simulink model "M2_chart_2"  (R2024a)
settings: Solver=FixedStepDiscrete  StartTime=0.0  StopTime=10.0  FixedStep=0.01  RelTol=1e-3  EnableMultiTasking=on
settings Model: Creator=saura  LastModifiedBy=Ishant
settings SolverCC: AlgebraicLoopSolver=TrustRegion  AutoInsertRateTranBlk=on
settings DataIOCC: LimitDataPoints=on
settings OptimizationCC: LifeSpan=inf
settings DebuggingCC: UnconnectedInputMsg=warning  UnconnectedOutputMsg=warning  UnconnectedLineMsg=warning  AllowSymbolicDim=off  SFUnexpectedBacktrackingDiag=warning  SFNoUnconditionalDefaultTransitionDiag=warning  SFExecutionAtInitializationDiag=none  ArithmeticOperatorsInVariantConditions=warning
settings ModelReferenceCC: EnableRefExpFcnMdlSchedulingChecks=on
settings SFSimCC: SimUseLocalCustomCode=off  CustomCodeUndefinedFunction=UseInterfaceOnly
settings RTWCC: RTWUseLocalCustomCode=off  GPUComputeCapability=3.5  DLArmComputeVersion=19.05
settings CodeAppCC: StateflowObjectComments=on
settings GRTTargetCC: TargetLangStandard=C89/C90 (ANSI)
settings ConfigComp: CovMetricSettings=dw  CovSaveCumulativeToWorkspaceVar=on  CovSaveSingleToWorkspaceVar=on  CovExternalEMLEnable=off  CovSFcnEnable=off

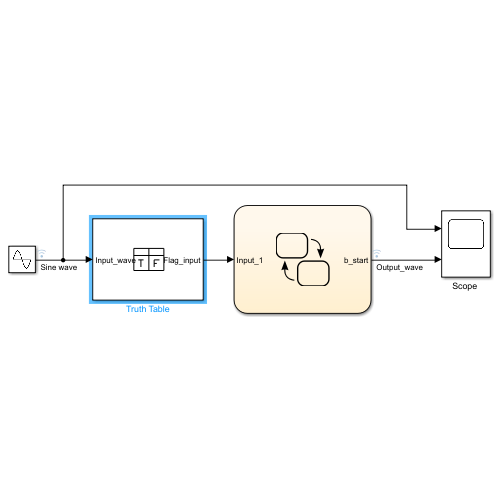
[thumbnail: Simulink's stored preview of the top-level diagram]
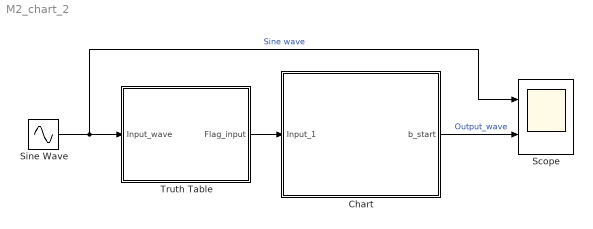
== system M2_chart_2 ==
  Chart : Stateflow chart  TreatAsAtomicUnit=on
  "Scope " : Scope  NumInputPorts=2
  Sine Wave : Sin  Amplitude=0.6
  Truth Table : Truth Table  TreatAsAtomicUnit=on
  wires:
  Sine Wave/1 -> "Scope "/1, Truth Table/1(Input_wave)  "Sine wave"
  Truth Table/1(Flag_input) -> Chart/1(Input_1)
  Chart/1(b_start) -> "Scope "/2  "Output_wave"

== matlab function M2_chart_2/Truth Table ==
  data: Input_wave input; Flag_input output
function Flag_input = fcn(Input_wave)

aVarTruthTableCondition_1 = false;
aVarTruthTableCondition_2 = false;


% condition2

aVarTruthTableCondition_1 = logical(Input_wave<=0.5);

% condition 1

aVarTruthTableCondition_2 = logical(Input_wave >0.5);

if (aVarTruthTableCondition_2)
    aFcnTruthTableAction_2();
elseif (aVarTruthTableCondition_1)
    aFcnTruthTableAction_1();
else % Default
    aFcnTruthTableAction_3();
end

function aFcnTruthTableAction_1()

% Example action 1 called from D2 column in condition table

Flag_input = 1;

function aFcnTruthTableAction_2()

% Example action 2 called from D1 column in condition table

Flag_input = -1

function aFcnTruthTableAction_3()

% nothing

Flag_input =0

== stateflow chart M2_chart_2/Chart ==
  state master
    state base [parallel]
      en:
      b_start=-1;
      settings: executionOrder=1
      state On [parallel]
        en:
        during:
        b_start=1;
        settings: executionOrder=1
      state Off [parallel]
        during:
        b_start=-1;
        settings: executionOrder=2
      (default) -> On
      Off -> On : [Input_1==-1]
      On -> Off : [Input_1==1]
    state double [parallel]
      during:
      output_sine_wave=2*input_sine_wave
      settings: executionOrder=2
    (default) -> double
  data: data local; b_start output double; Input_1 input double
